simulink model "fixed_point"  (R2022b)
settings: Solver=VariableStepAuto  StartTime=0.0  StopTime=1000.0  RelTol=1e-3
settings Model: Creator=Вячеслав  LastModifiedBy=Вячеслав

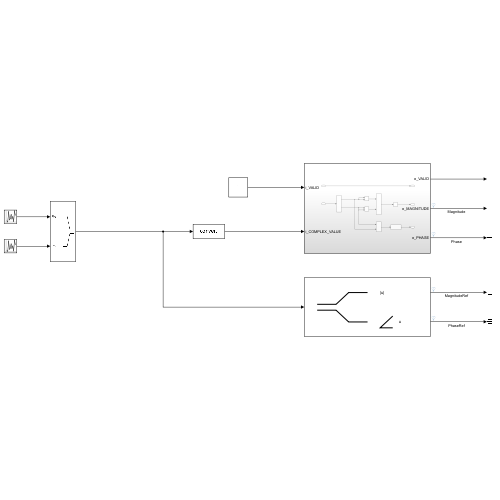
[thumbnail: Simulink's stored preview of the top-level diagram]
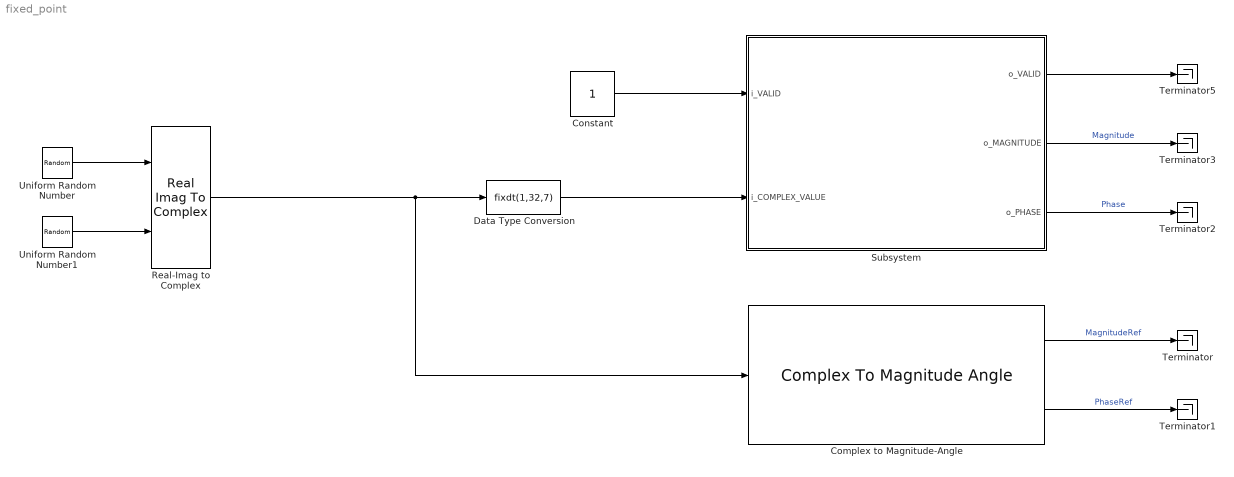
== system fixed_point ==
  Complex to Magnitude-Angle : ComplexToMagnitudeAngle
  Constant : Constant  OutDataTypeStr=boolean  SampleTime=-1
  Data Type Conversion : DataTypeConversion  OutDataTypeStr=fixdt(1,32,7)  RndMeth=Round  SaturateOnIntegerOverflow=off
  Real-Imag to Complex : RealImagToComplex
  Subsystem : Subsystem
  Terminator{,1..3,5} (5 alike) : Terminator
  Uniform Random Number : UniformRandomNumber  Minimum=-2^(25-1)  Maximum=2^(25-1)-1/2^7  Seed=25  SampleTime=1
  Uniform Random Number1 : UniformRandomNumber  Minimum=-2^(25-1)  Maximum=2^(25-1)-1/2^7  Seed=26  SampleTime=1
  wires:
  Data Type Conversion/1 -> Subsystem/2(i_COMPLEX_VALUE)
  Subsystem/1(o_VALID) -> Terminator5/1
  Subsystem/3(o_PHASE) -> Terminator2/1  "Phase"
  Subsystem/2(o_MAGNITUDE) -> Terminator3/1  "Magnitude"
  Complex to Magnitude-Angle/2 -> Terminator1/1  "PhaseRef"
  Complex to Magnitude-Angle/1 -> Terminator/1  "MagnitudeRef"
  Constant/1 -> Subsystem/1(i_VALID)
  Real-Imag to Complex/1 -> Data Type Conversion/1, Complex to Magnitude-Angle/1
  Uniform Random Number/1 -> Real-Imag to Complex/1
  Uniform Random Number1/1 -> Real-Imag to Complex/2

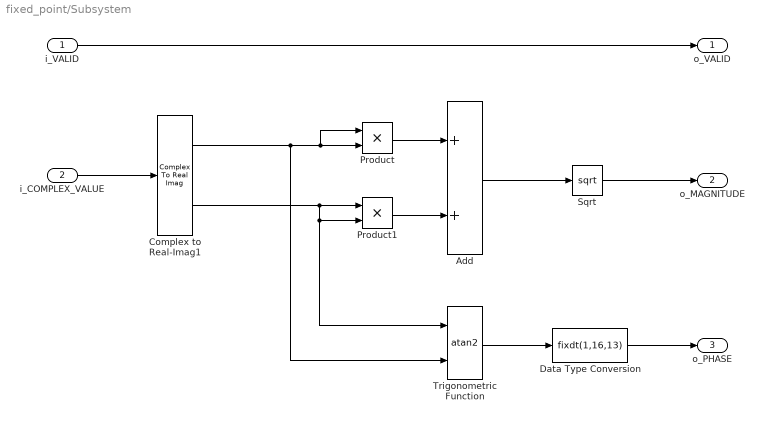
== system fixed_point/Subsystem ==
  i_VALID : Inport  OutDataTypeStr=boolean
  i_COMPLEX_VALUE : Inport  Port=2  LockScale=on
  Add : Sum
  Complex to Real-Imag1 : ComplexToRealImag
  Data Type Conversion : DataTypeConversion  OutDataTypeStr=fixdt(1,16,13)  RndMeth=Round  SaturateOnIntegerOverflow=off
  Product : Product
  Product1 : Product
  Sqrt : Sqrt  OutDataTypeStr=fixdt(1,33,7)
  Trigonometric Function : Trigonometry  Operator=atan2  ApproximationMethod=CORDIC
  o_VALID : Outport  OutDataTypeStr=boolean
  o_MAGNITUDE : Outport  Port=2
  o_PHASE : Outport  Port=3
  wires:
  i_VALID/1 -> o_VALID/1
  Complex to Real-Imag1/1 -> Trigonometric Function/2, Product/1, Product/2
  i_COMPLEX_VALUE/1 -> Complex to Real-Imag1/1
  Add/1 -> Sqrt/1
  Complex to Real-Imag1/2 -> Trigonometric Function/1, Product1/2, Product1/1
  Product1/1 -> Add/2
  Product/1 -> Add/1
  Trigonometric Function/1 -> Data Type Conversion/1
  Data Type Conversion/1 -> o_PHASE/1
  Sqrt/1 -> o_MAGNITUDE/1
